simulink subsystem "PieroModel"  (R2023b)
settings: Solver=VariableStepAuto  StartTime=0.0  StopTime=10.0  RelTol=1e-3
settings Model: Creator=juana  LastModifiedBy=juana

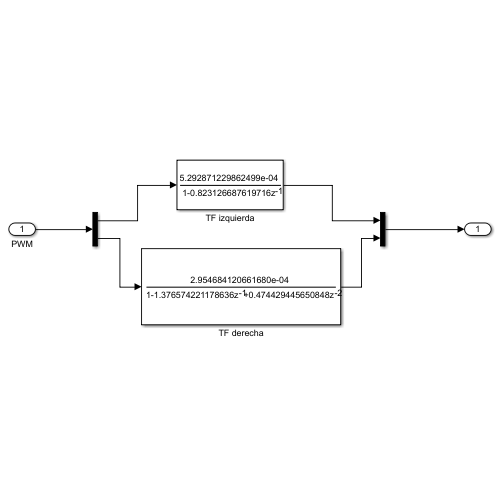
[thumbnail: Simulink's stored preview of the top-level diagram]
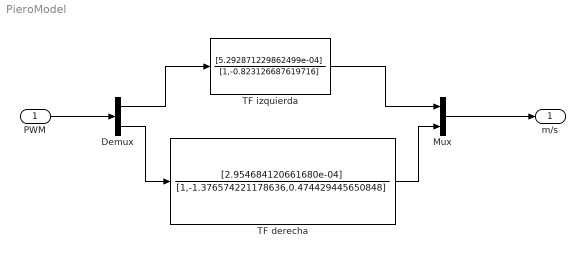
== system PieroModel ==
  PWM : Inport  OutMin=[-255]  OutMax=[255]
  Demux : Demux  Outputs=2
  Mux : Mux  Inputs=2
  TF derecha : DiscreteFilter  Numerator=[2.954684120661680e-04]  Denominator=[1,-1.376574221178636,0.474429445650848]
  TF izquierda : DiscreteFilter  Numerator=[5.292871229862499e-04]  Denominator=[1,-0.823126687619716]
  m/s : Outport
  wires:
  Mux/1 -> m/s/1
  PWM/1 -> Demux/1
  Demux/1 -> TF izquierda/1
  TF izquierda/1 -> Mux/1
  Demux/2 -> TF derecha/1
  TF derecha/1 -> Mux/2
